simulink model "rover_bot_obstacles"  (R2021a)
settings: Solver=ode23t  StartTime=0.0  StopTime=60  RelTol=1e-3
model workspace (MATLAB code in the model file):
  | a=3;
  | SplinePoints=[-a, -a
  |     -0.904*a, -1.019*a,
  |     -0.8*a, -a
  |     0, -0.9*a
  |     a, -a
  |     0.9*a, 0
  |     a, a
  |     0, 0.9*a
  |     -a, a
  |     -0.9*a, 0
  |     -a, -0.8*a
  |     -1.019*a, -0.904*a];
values from neighbouring files (symbols this model uses):
  m = size(mapxy,1)    [distance2curveSimplified.m]
undefined symbols (not defined in the file or in its folder): distance2curveKH, X, Y, Z
libraries: sm_lib x42, nesl_utility x16
(part 1 of 2)
settings Model: Creator=kjartan  LastModifiedBy=kjartan

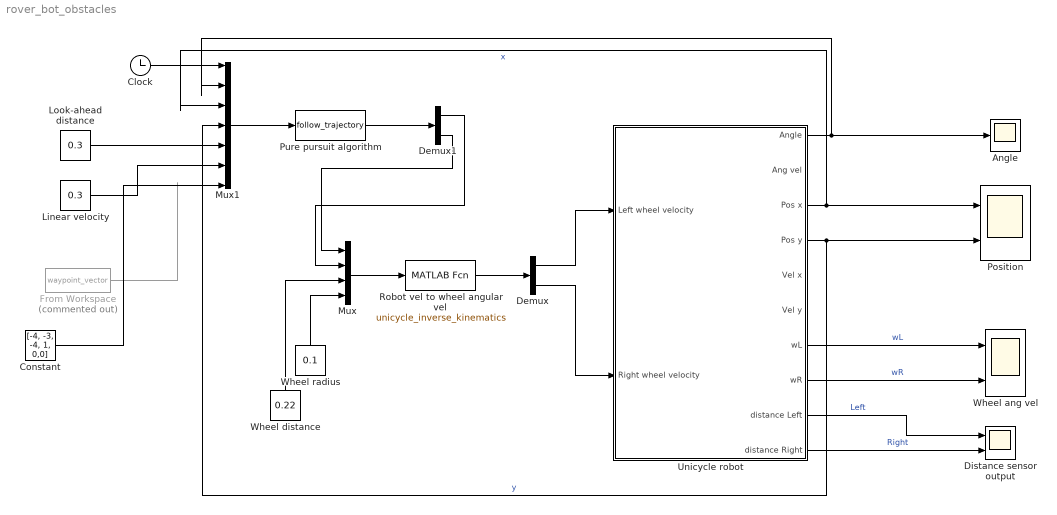
== system rover_bot_obstacles ==
  Angle : Scope
  Clock : Clock
  Constant : Constant  Value=[-4, -3, -4, 1, 0,0]
  Demux : Demux  Outputs=2
  Demux1 : Demux  Outputs=2
  Distance sensor output : Scope  NumInputPorts=2
  From Workspace : FromWorkspace  Commented=on  VariableName=waypoint_vector
  Linear velocity : Constant  Value=0.3
  Look-ahead distance : Constant  Value=0.3
  Mux : Mux
  Mux1 : Mux  Inputs=7
  Position : Scope  NumInputPorts=2
  Pure pursuit algorithm : MATLABFcn  MATLABFcn=follow_trajectory  OutputDimensions=2
  Robot vel to wheel angular vel : MATLABFcn  MATLABFcn=unicycle_inverse_kinematics  OutputDimensions=2
  Unicycle robot : Subsystem
  Wheel ang vel : Scope  NumInputPorts=2
  Wheel distance : Constant  Value=0.22
  Wheel radius : Constant  Value=0.1
  wires:
  Unicycle robot/3(Pos x) -> Mux1/3, Position/1  "x"
  Unicycle robot/4(Pos y) -> Mux1/4, Position/2  "y"
  Unicycle robot/7(wL) -> Wheel ang vel/1  "wL"
  Unicycle robot/8(wR) -> Wheel ang vel/2  "wR"
  Unicycle robot/1(Angle) -> Mux1/2, Angle/1
  Unicycle robot/9(distance Left) -> Distance sensor output/1  "Left"
  Unicycle robot/10(distance Right) -> Distance sensor output/2  "Right"
  Robot vel to wheel angular vel/1 -> Demux/1
  Demux/1 -> Unicycle robot/1(Left wheel velocity)
  Mux/1 -> Robot vel to wheel angular vel/1
  Wheel distance/1 -> Mux/3
  Wheel radius/1 -> Mux/4
  Demux1/1 -> Mux/2
  Demux/2 -> Unicycle robot/2(Right wheel velocity)
  Mux1/1 -> Pure pursuit algorithm/1
  Pure pursuit algorithm/1 -> Demux1/1
  Demux1/2 -> Mux/1
  Clock/1 -> Mux1/1
  From Workspace/1 -> ?
  Look-ahead distance/1 -> Mux1/5
  Linear velocity/1 -> Mux1/6
  Constant/1 -> Mux1/7
